simulink model "gm_sampleModel61706_pp_36_1_sub"  (R2023b)
settings: Solver=VariableStepAuto  StartTime=0.0  StopTime=10.0  RelTol=1e-3
libraries: simulink x39, hdlsllib x2
(part 1 of 2)
settings Model: Creator=CW  LastModifiedBy=CW
settings OptimizationCC: BlockReduction=off  ConditionallyExecuteInputs=off
settings DebuggingCC: ArtificialAlgebraicLoopMsg=none  InheritedTsInSrcMsg=none

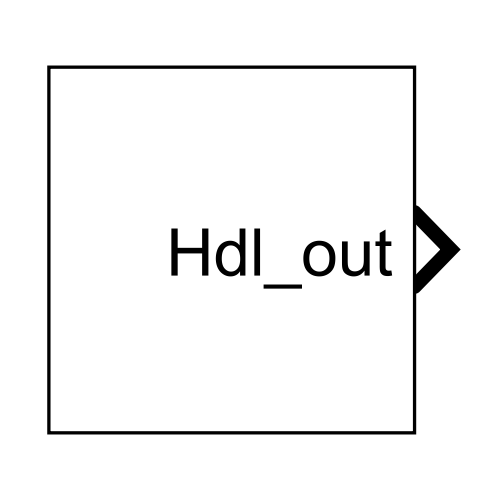
[thumbnail: Simulink's stored preview of the top-level diagram]
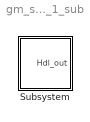
== system gm_sampleModel61706_pp_36_1_sub ==
  Subsystem : Subsystem

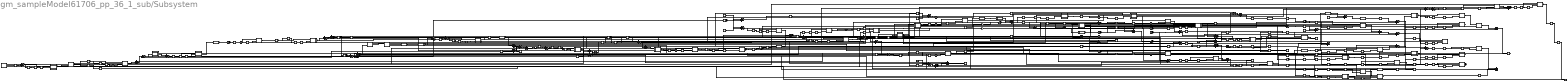
== system gm_sampleModel61706_pp_36_1_sub/Subsystem ==
  Reshape{,1..8} (9 alike) : Reshape
  cfblk1 : Constant  Value=0  OutDataTypeStr=uint8  SampleTime=1
  cfblk10 : Subsystem
  cfblk{11,14..15,20,31,34,39,41,47..48,54,56,58,73,87,90..91,94..95,100,111,118..119,122,125,127,130,133..134,138,141,158,169,178} (34 alike) : Sum  OutDataTypeStr=uint8  AccumDataTypeStr=uint8  SampleTime=1
  cfblk{26,101,110,148,166,168,184} (7 alike) : MinMax  OutDataTypeStr=uint8
  cfblk102 : Subsystem
  cfblk103 : Subsystem
  cfblk{18,42,51,79,84,104,120,132,136,147,153,165} (12 alike) : Product  Inputs=*/  OutDataTypeStr=uint8  RndMeth=Zero  SaturateOnIntegerOverflow=on  SampleTime=1
  cfblk105 : Subsystem
  cfblk106_inst : Subsystem
  cfblk{17,19,40,44,59,62,83,107..108,112,114,159,180,183} (14 alike) : Sum  Inputs=+-  OutDataTypeStr=uint8  AccumDataTypeStr=uint8  SampleTime=1
  cfblk{21,25,52,65,75,93,109,115,124,151,163,167} (12 alike) : Sum  Inputs=+  OutDataTypeStr=uint8
  cfblk{23,29..30,43,53,113} (6 alike) : Gain  Gain="fi(0,0,8,7,\"hex\",\"80\")"  ParamDataTypeStr=fixdt(0, 8, 7)  OutDataTypeStr=uint8  SampleTime=1
  cfblk116 : Subsystem
  cfblk117 : Subsystem
  cfblk12 : Subsystem
  cfblk123 : Subsystem
  cfblk126 : Subsystem
  cfblk129 : Subsystem
  cfblk13 : Subsystem  mask(Real World Value Increment){}
      mask help: Simulink:masks:RealWorldValueIncrement_MD
      mask Display: disp('V++')
  cfblk{24,63,131,142..144,149,152} (8 alike) : Abs  SampleTime=1  OutDataTypeStr=uint8  SaturateOnIntegerOverflow=off
  cfblk{69,92,135,140,160} (5 alike) : Signum  SampleTime=1
  cfblk{27,36,67..68,137,156,170..171,175} (9 alike) : Sum  OutDataTypeStr=uint8  AccumDataTypeStr=uint8  RndMeth=Nearest  SampleTime=1
  cfblk137_const_val : Constant  Value=0  VectorParams1D=off  OutDataTypeStr=uint8  SampleTime=1
  cfblk139_inst : Subsystem
  cfblk145 : Subsystem
  cfblk146_inst : Subsystem
  cfblk150_inst : Subsystem
  cfblk{22,33,78,154} (4 alike) : ComplexToRealImag  SampleTime=1
  cfblk155 : Subsystem
  cfblk156_const_val : Constant  Value=0  VectorParams1D=off  OutDataTypeStr=uint8  SampleTime=1
  cfblk157_inst : Subsystem
  cfblk16 : Subsystem
  cfblk161 : Subsystem
  cfblk162_inst : Subsystem
  cfblk164 : Subsystem
  cfblk170_const_val : Constant  Value=0  VectorParams1D=off  OutDataTypeStr=uint8  SampleTime=1
  cfblk171_const_val : Constant  Value=0  VectorParams1D=off  OutDataTypeStr=uint8  SampleTime=1
  cfblk172_inst : Subsystem
  cfblk174 : Subsystem
  cfblk175_const_val : Constant  Value=0  VectorParams1D=off  OutDataTypeStr=uint8  SampleTime=1
  cfblk176 : Subsystem
  cfblk179 : Subsystem
  cfblk182 : Subsystem  mask(Real World Value Increment){}
      mask help: Simulink:masks:RealWorldValueIncrement_MD
      mask Display: disp('V++')
  cfblk185 : Constant  Value=double(0)  VectorParams1D=off  OutDataTypeStr=double  SampleTime=1
  cfblk186 : hdlsllib/Sources/HDL Counter  CountType=Count limited  CountInit=0  CountStep=1  CountMax=25  CountFromType=Initial value  CountFrom=0  CountResetPort=off  CountLoadPort=off  CountEnbPort=off  CountDirPort=off  CountHitOutputPort=off  CountDataType=Unsigned  CountWordLen=8  CountFracLen=0  CountSampTime=1
  cfblk187 : Constant  OutDataTypeStr=uint8  SampleTime=1
  cfblk188 : Subsystem
  cfblk189 : Subsystem
  cfblk190 : Switch  Threshold=double(0)  OutDataTypeStr=uint8  SampleTime=1  SaturateOnIntegerOverflow=off  InputSameDT=off
  cfblk191 : Switch  Threshold=double(0)  OutDataTypeStr=uint8  SampleTime=1  SaturateOnIntegerOverflow=off  InputSameDT=off
  cfblk192 : Switch  Threshold=double(0)  OutDataTypeStr=uint8  SampleTime=1  SaturateOnIntegerOverflow=off  InputSameDT=off
  cfblk{193..196,198..199,201..215,217} (22 alike) : Delay  DelayLength=double(2)  InitialCondition=0  SampleTime=1
  cfblk197 : Subsystem
  cfblk2 : Subsystem  mask(Compare To Constant){relop=<=, const=double(3), OutDataTypeStr=uint8, ZeroCross=on}
      mask prompts: relop "Simulink:masks:Operator_MP"; const "Simulink:masks:ConstantValue_MP"; OutDataTypeStr "Simulink:masks:OutputDataType_MP"; ZeroCross "Simulink:masks:EnableZerocrossingDetection_MP"
      mask help: Simulink:masks:CompareToConstant_MD
      mask init:
      | OutDataTypeStr = 'uint8';
      | ZeroCross = 'on';
      | blkName = 'sampleModel61706_pp_36_1_sub/Subsystem/cfblk2';
      | const = double(3);
      | const_str = '3.0';
      | const_val = double(3);
      | relop = '<=';
      | setValue = 'fixdt(0, 8)';
      | str = '<= 3';
      mask TypeOptions relop: == | ~= | < | <= | >= | >
      mask TypeOptions OutDataTypeStr: Simulink:masks:uint8 | Simulink:masks:boolean
      mask Callback ZeroCross: sl('zeroCrossEnable', gcbh);
      mask Display: disp(str)
  cfblk200 : Subsystem
  cfblk218 : Subsystem
  cfblk219 : DataTypeConversion  OutDataTypeStr=fixdt(0,8,0)
  cfblk27_const_val : Constant  Value=0  VectorParams1D=off  OutDataTypeStr=uint8  SampleTime=1
  cfblk28 : Subsystem
  cfblk3 : Subsystem
  cfblk32 : Subsystem
  cfblk36_const_val : Constant  Value=0  VectorParams1D=off  OutDataTypeStr=uint8  SampleTime=1
  cfblk37 : Subsystem
  cfblk38 : Subsystem
  cfblk4 : Subsystem  mask(Compare To Zero){relop=<=, OutDataTypeStr=uint8, ZeroCross=on}
      mask prompts: relop "Simulink:masks:Operator_MP"; OutDataTypeStr "Simulink:masks:OutputDataType_MP"; ZeroCross "Simulink:masks:EnableZerocrossingDetection_MP"
      mask help: Simulink:masks:CompareToZero_MD
      mask init:
      | OutDataTypeStr = 'uint8';
      | ZeroCross = 'on';
      | blkName = 'sampleModel61706_pp_36_1_sub/Subsystem/cfblk4';
      | relop = '<=';
      | setValue = 'fixdt(0, 8)';
      mask TypeOptions relop: == | ~= | < | <= | >= | >
      mask TypeOptions OutDataTypeStr: Simulink:masks:uint8 | Simulink:masks:boolean
      mask Callback ZeroCross: sl('zeroCrossEnable', gcbh);
      mask Display: disp([relop,' 0'])
  cfblk45_inst : Subsystem
  cfblk49 : Subsystem
  cfblk5 : Subsystem  mask(Compare To Constant){relop=<=, const=double(3), OutDataTypeStr=uint8, ZeroCross=on}
      mask prompts: relop "Simulink:masks:Operator_MP"; const "Simulink:masks:ConstantValue_MP"; OutDataTypeStr "Simulink:masks:OutputDataType_MP"; ZeroCross "Simulink:masks:EnableZerocrossingDetection_MP"
      mask help: Simulink:masks:CompareToConstant_MD
      mask init:
      | OutDataTypeStr = 'uint8';
      | ZeroCross = 'on';
      | blkName = 'sampleModel61706_pp_36_1_sub/Subsystem/cfblk5';
      | const = double(3);
      | const_str = '3.0';
      | const_val = double(3);
      | relop = '<=';
      | setValue = 'fixdt(0, 8)';
      | str = '<= 3';
      mask TypeOptions relop: == | ~= | < | <= | >= | >
      mask TypeOptions OutDataTypeStr: Simulink:masks:uint8 | Simulink:masks:boolean
      mask Callback ZeroCross: sl('zeroCrossEnable', gcbh);
      mask Display: disp(str)
  cfblk50 : Sum  OutDataTypeStr=uint8  AccumDataTypeStr=fixdt(0, 32, 7)  SampleTime=1
  cfblk55 : Subsystem
  cfblk57 : Subsystem
  cfblk60 : Subsystem  mask(Real World Value Increment){}
      mask help: Simulink:masks:RealWorldValueIncrement_MD
      mask Display: disp('V++')
  cfblk64 : Subsystem
  cfblk66 : Subsystem
  cfblk67_const_val : Constant  Value=0  VectorParams1D=off  OutDataTypeStr=uint8  SampleTime=1
  cfblk68_const_val : Constant  Value=0  VectorParams1D=off  OutDataTypeStr=uint8  SampleTime=1
  cfblk6_inst : Subsystem
  cfblk7 : Subsystem
  cfblk70 : Subsystem  mask(Real World Value Increment){}
      mask help: Simulink:masks:RealWorldValueIncrement_MD
      mask Display: disp('V++')
  cfblk71_inst : Subsystem
  cfblk72 : Subsystem  mask(Real World Value Increment){}
      mask help: Simulink:masks:RealWorldValueIncrement_MD
      mask Display: disp('V++')
  cfblk74 : Subsystem
  cfblk76 : Subsystem
  cfblk77 : Sum  OutDataTypeStr=uint8  AccumDataTypeStr=fixdt(0, 32, 7)  SampleTime=1
  cfblk8 : Subsystem
  cfblk80 : Subsystem  mask(Real World Value Increment){}
      mask help: Simulink:masks:RealWorldValueIncrement_MD
      mask Display: disp('V++')
  cfblk81 : Subsystem  mask(Real World Value Increment){}
      mask help: Simulink:masks:RealWorldValueIncrement_MD
      mask Display: disp('V++')
  cfblk85 : Sum  OutDataTypeStr=uint8  AccumDataTypeStr=fixdt(0, 32, 7)  SampleTime=1
  cfblk86_inst : Subsystem
  cfblk88 : Gain  Gain="fi(0,0,16,15,\"hex\",\"8000\")"  ParamDataTypeStr=fixdt(0, 16, 15)  OutDataTypeStr=uint8  SampleTime=1
  cfblk89 : Subsystem
  cfblk9 : Subsystem  mask(Real World Value Increment){}
      mask help: Simulink:masks:RealWorldValueIncrement_MD
      mask Display: disp('V++')
  cfblk96 : Subsystem
  cfblk97_inst : Subsystem
  cfblk98 : Subsystem
  cfblk99 : Subsystem
  compare{,1,8..11,14,16..19,23,25,27..28,32..37} (21 alike) : simulink/Logic and Bit Operations/Compare To Constant  relop=>=  const=255  OutDataTypeStr=boolean
  compare{2,4..7,12..13,15,20,22,24,26,29..31} (15 alike) : simulink/Logic and Bit Operations/Compare To Constant  relop=>=  const=0  OutDataTypeStr=boolean
  compare21 : simulink/Logic and Bit Operations/Compare To Constant  relop=>=  const=1  OutDataTypeStr=boolean
  compare3 : simulink/Logic and Bit Operations/Compare To Constant  relop=>=  const=1  OutDataTypeStr=boolean
  compare38 : simulink/Logic and Bit Operations/Compare To Constant  relop=>=  const=1  OutDataTypeStr=boolean
  emi_{6,14,22,30,39,47,55,63,71,79,87,95,103,111,119,127,136,144,152,160,176,184,192,200,208,216,224,232,240,256,264,272,280,288,296,304,312} (37 alike) : DataTypeConversion  OutDataTypeStr=fixdt(0,8,0)
  emi_{7,56,64,72,80,88,104,112,161,169,177,185,209,217,225,233,241,273,289,297,305} (21 alike) : Delay  DelayLength=double(2)  InitialCondition=255  SampleTime=1
  emi_{15,23,31,40,48,120,137,145,153,193,201,249,265,281,313} (15 alike) : Delay  DelayLength=double(2)  InitialCondition=0  SampleTime=1
  emi_128 : Delay  DelayLength=double(2)  InitialCondition=1  SampleTime=1
  emi_168 : DataTypeConversion  OutDataTypeStr=uint8  SampleTime=1  SaturateOnIntegerOverflow=off  RndMeth=Floor
  emi_248 : DataTypeConversion  OutDataTypeStr=uint8  SampleTime=1  SaturateOnIntegerOverflow=off  RndMeth=Floor
  emi_257 : Delay  DelayLength=double(2)  InitialCondition=1  SampleTime=1
  emi_96 : Delay  DelayLength=double(2)  InitialCondition=1  SampleTime=1
  Hdl_out : Outport  OutDataTypeStr=uint8  SampleTime=1
  wires:
  cfblk1/1 -> cfblk114/1
  cfblk10/1(emi_2) -> cfblk206/1
  cfblk100/1 -> cfblk22/1, cfblk165/1
  cfblk101/1 -> emi_161/1, cfblk3/1(emi_155)
  cfblk102/1(emi_10) -> cfblk130/1
  cfblk103/1(emi_115) -> cfblk120/1
  cfblk104/1 -> emi_185/1, cfblk38/1(emi_179), cfblk120/2
  cfblk105/1(emi_276) -> cfblk63/1, cfblk34/2
  cfblk106_inst/1(out1) -> cfblk135/1, cfblk25/1
  cfblk107/1 -> cfblk211/1
  cfblk108/1 -> cfblk188/1(In1)
  cfblk109/1 -> cfblk178/2, cfblk134/1
  cfblk11/1 -> emi_104/1, cfblk161/1(emi_98)
  cfblk110/1 -> cfblk41/2, cfblk137/1
  cfblk111/1 -> cfblk100/1, emi_80/1, cfblk145/1(emi_74)
  cfblk112/1 -> cfblk90/1, Hdl_out/1
  cfblk113/1 -> emi_145/1, cfblk218/1(emi_139)
  cfblk114/1 -> cfblk133/1
  cfblk115/1 -> cfblk192/3, emi_201/1, cfblk49/1(emi_195)
  cfblk116/1(emi_18) -> cfblk30/1
  cfblk117/1(emi_26) -> emi_281/1, cfblk105/1(emi_275)
  cfblk118/1 -> cfblk59/1
  cfblk119/1 -> cfblk62/1
  cfblk12/1(emi_34) -> cfblk160/1
  cfblk12/2(emi_35) -> cfblk136/2, cfblk79/2
  cfblk120/1 -> cfblk54/2, emi_88/1, cfblk155/1(emi_82)
  Reshape/1 -> cfblk191/1
  cfblk122/1 -> cfblk169/1
  cfblk123/1(emi_43) -> cfblk142/1
  cfblk124/1 -> cfblk19/1
  cfblk125/1 -> emi_56/1, cfblk126/1(emi_50)
  cfblk126/1(emi_51) -> cfblk50/1
  cfblk127/1 -> cfblk6_inst/1(in1)
  Reshape1/1 -> cfblk67/1
  cfblk129/1(emi_59) -> cfblk111/1
  cfblk13/1(y) -> cfblk154/1
  cfblk130/1 -> emi_40/1, cfblk12/1(emi_33)
  cfblk131/1 -> cfblk189/1(In1)
  cfblk132/1 -> cfblk203/1
  cfblk133/1 -> cfblk71_inst/1(in1), cfblk56/2
  cfblk134/1 -> cfblk107/1
  cfblk135/1 -> emi_112/1, cfblk164/1(emi_106)
  cfblk136/1 -> cfblk208/1, cfblk207/1
  cfblk137/1 -> cfblk209/1
  cfblk138/1 -> emi_225/1, cfblk200/1(emi_219)
  cfblk139_inst/1(out1) -> cfblk182/1(u)
  cfblk14/1 -> emi_193/1, cfblk176/1(emi_187)
  cfblk140/1 -> cfblk56/1, cfblk112/1
  cfblk141/1 -> cfblk36/1, cfblk100/2
  cfblk142/1 -> cfblk83/2, cfblk23/1
  cfblk143/1 -> cfblk150_inst/1(in1), cfblk134/2, cfblk111/2
  cfblk144/1 -> cfblk153/2
  cfblk145/1(emi_75) -> emi_7/1, cfblk10/1(emi_1)
  cfblk146_inst/1(out1) -> emi_273/1, cfblk197/1(emi_267)
  cfblk147/1 -> cfblk85/1, cfblk131/1
  cfblk148/1 -> emi_257/1, cfblk76/1(emi_251)
  cfblk149/1 -> emi_241/1, cfblk7/1(emi_235)
  cfblk15/1 -> emi_15/1, cfblk102/1(emi_9)
  cfblk150_inst/1(out1) -> cfblk166/1
  cfblk151/1 -> cfblk143/1, cfblk108/1
  cfblk152/1 -> cfblk73/1, cfblk41/1, cfblk162_inst/1(in1)
  cfblk153/1 -> cfblk11/1
  cfblk154/1 -> cfblk58/1
  cfblk154/2 -> Reshape2/1, cfblk80/1(u)
  cfblk155/1(emi_83) -> cfblk190/1, cfblk17/1
  cfblk156/1 -> cfblk2/1(u)
  cfblk157_inst/1(out1) -> cfblk44/2, cfblk202/1
  cfblk158/1 -> cfblk21/1
  cfblk159/1 -> cfblk157_inst/2(in2), cfblk204/1
  cfblk16/1(emi_91) -> cfblk77/1
  cfblk160/1 -> cfblk70/1(u)
  cfblk161/1(emi_99) -> cfblk68/1, cfblk17/2
  cfblk162_inst/1(out1) -> cfblk180/1
  cfblk163/1 -> cfblk180/2
  cfblk164/1(emi_107) -> cfblk119/2
  cfblk165/1 -> cfblk59/2
  cfblk166/1 -> cfblk91/1, cfblk26/1
  cfblk167/1 -> cfblk152/1, cfblk42/2
  cfblk168/1 -> cfblk39/1
  cfblk169/1 -> cfblk171/1
  cfblk17/1 -> cfblk192/2
  cfblk170/1 -> cfblk79/1
  cfblk171/1 -> cfblk115/1
  cfblk172_inst/1(out1) -> cfblk139_inst/1(in1)
  Reshape2/1 -> emi_120/1, cfblk103/1(emi_114)
  cfblk174/1(emi_123) -> cfblk47/1
  cfblk175/1 -> Reshape/1
  cfblk176/1(emi_188) -> cfblk95/1
  Reshape3/1 -> cfblk110/1
  cfblk178/1 -> emi_31/1, cfblk117/1(emi_25), cfblk124/1
  cfblk179/1(emi_131) -> Reshape5/1
  cfblk179/2(emi_132) -> cfblk146_inst/1(in1), cfblk198/1
  cfblk18/1 -> cfblk45_inst/1(in1), cfblk93/1
  cfblk180/1 -> emi_217/1, cfblk57/1(emi_211)
  Reshape4/1 -> emi_23/1, cfblk53/1, cfblk116/1(emi_17)
  cfblk182/1(y) -> cfblk81/1(u)
  cfblk183/1 -> emi_48/1, cfblk123/1(emi_42)
  cfblk184/1 -> emi_289/1, cfblk89/1(emi_283)
  cfblk185/1 -> cfblk72/1(u)
  cfblk186/1 -> cfblk50/2, cfblk183/1, cfblk14/1
  cfblk187/1 -> Reshape7/1, cfblk107/2
  cfblk188/1(Out1) -> cfblk125/2, cfblk212/1
  cfblk189/1(Out1) -> cfblk94/2
  cfblk19/1 -> cfblk151/1
  cfblk190/1 -> cfblk122/2, emi_137/1, cfblk199/1, cfblk179/1(emi_130)
  cfblk191/1 -> cfblk158/1
  cfblk192/1 -> cfblk194/1
  cfblk193/1 -> cfblk119/1
  cfblk194/1 -> cfblk51/2
  cfblk195/1 -> cfblk191/3
  cfblk196/1 -> cfblk62/2
  cfblk197/1(emi_268) -> cfblk158/2
  cfblk198/1 -> cfblk114/2
  cfblk199/1 -> cfblk87/2
  cfblk2/1(y) -> cfblk69/1
  cfblk20/1 -> cfblk165/2, cfblk148/1
  cfblk200/1(emi_220) -> cfblk190/3
  cfblk201/1 -> cfblk84/2
  cfblk202/1 -> cfblk150_inst/2(in2)
  cfblk203/1 -> cfblk127/1
  cfblk204/1 -> cfblk130/2
  cfblk205/1 -> cfblk18/1
  cfblk206/1 -> cfblk85/2
  cfblk207/1 -> cfblk19/2
  cfblk208/1 -> cfblk71_inst/2(in2)
  cfblk209/1 -> cfblk191/2
  cfblk21/1 -> cfblk5/1(u)
  cfblk210/1 -> cfblk15/2
  cfblk211/1 -> cfblk122/1
  cfblk212/1 -> cfblk106_inst/1(in1)
  cfblk213/1 -> cfblk31/2
  cfblk214/1 -> cfblk169/2
  cfblk215/1 -> cfblk147/2
  cfblk217/1 -> cfblk133/2
  cfblk218/1(emi_140) -> cfblk31/1, cfblk172_inst/1(in1)
  cfblk219/1 -> cfblk113/1
  cfblk22/1 -> cfblk140/1
  cfblk22/2 -> cfblk92/1
  cfblk23/1 -> emi_153/1, cfblk43/1, cfblk64/1(emi_147)
  cfblk24/1 -> cfblk75/1
  cfblk25/1 -> cfblk217/1
  cfblk26/1 -> cfblk91/2, cfblk20/2
  cfblk27/1 -> cfblk108/2, emi_177/1, cfblk37/1(emi_171)
  cfblk28/1(emi_67) -> cfblk215/1, cfblk104/1
  cfblk29/1 -> cfblk109/1
  cfblk3/1(emi_156) -> cfblk159/2, cfblk141/2
  cfblk30/1 -> cfblk9/1(u)
  cfblk31/1 -> cfblk15/1
  cfblk32/1(emi_164) -> cfblk88/1
  cfblk33/1 -> cfblk147/1
  cfblk33/2 -> cfblk13/1(u)
  cfblk34/1 -> emi_64/1, cfblk129/1(emi_58)
  Reshape5/1 -> cfblk48/2, cfblk170/1
  cfblk36/1 -> cfblk138/2, cfblk118/2
  cfblk37/1(emi_172) -> cfblk94/1
  cfblk38/1(emi_180) -> cfblk58/2
  cfblk39/1 -> cfblk153/1
  cfblk4/1(y) -> cfblk178/1
  cfblk40/1 -> cfblk193/1
  cfblk41/1 -> cfblk95/2, cfblk44/1
  cfblk42/1 -> cfblk138/1, emi_305/1, cfblk210/1, cfblk98/1(emi_299)
  cfblk43/1 -> emi_265/1, cfblk8/1(emi_259)
  cfblk44/1 -> cfblk201/1
  cfblk45_inst/1(out1) -> emi_297/1, cfblk96/1(emi_291)
  Reshape6/1 -> cfblk136/1, cfblk52/1
  cfblk47/1 -> cfblk90/2
  cfblk48/1 -> cfblk118/1, cfblk196/1
  cfblk49/1(emi_196) -> Reshape8/1, cfblk14/2, cfblk139_inst/2(in2)
  cfblk5/1(y) -> cfblk219/1
  cfblk50/1 -> cfblk213/1
  cfblk51/1 -> cfblk146_inst/2(in2), cfblk125/1, cfblk18/2
  cfblk52/1 -> cfblk47/2
  cfblk53/1 -> cfblk104/2
  cfblk54/1 -> cfblk34/1
  cfblk55/1(emi_204) -> emi_72/1, cfblk28/1(emi_66)
  cfblk56/1 -> cfblk205/1
  cfblk57/1(emi_212) -> cfblk60/1(u)
  cfblk58/1 -> cfblk45_inst/2(in2), cfblk184/1
  cfblk59/1 -> cfblk144/1
  cfblk6_inst/1(out1) -> emi_209/1, cfblk55/1(emi_203)
  cfblk60/1(y) -> cfblk54/1, cfblk149/1
  Reshape7/1 -> emi_96/1, cfblk16/1(emi_90)
  cfblk62/1 -> cfblk162_inst/2(in2), cfblk65/1
  cfblk63/1 -> emi_313/1, cfblk99/1(emi_307)
  cfblk64/1(emi_148) -> emi_249/1, cfblk74/1(emi_243)
  cfblk65/1 -> cfblk27/1, cfblk175/1
  cfblk66/1(emi_228) -> cfblk97_inst/2(in2), cfblk106_inst/2(in2)
  cfblk67/1 -> cfblk40/2, cfblk39/2
  cfblk68/1 -> cfblk192/1
  cfblk69/1 -> cfblk20/1
  cfblk7/1(emi_236) -> cfblk101/1
  cfblk70/1(y) -> cfblk48/1, cfblk51/1
  cfblk71_inst/1(out1) -> cfblk33/1, Reshape4/1
  cfblk72/1(y) -> cfblk4/1(u)
  cfblk73/1 -> Reshape3/1
  cfblk74/1(emi_244) -> cfblk77/2
  cfblk75/1 -> cfblk157_inst/1(in1)
  cfblk76/1(emi_252) -> cfblk141/1
  cfblk77/1 -> emi_128/1, cfblk174/1(emi_122)
  cfblk78/1 -> cfblk168/1
  cfblk78/2 -> cfblk24/1, cfblk132/2
  cfblk79/1 -> cfblk195/1
  cfblk8/1(emi_260) -> cfblk97_inst/1(in1)
  cfblk80/1(y) -> cfblk156/1
  cfblk81/1(y) -> cfblk159/1, cfblk132/1
  Reshape8/1 -> cfblk29/1
  cfblk83/1 -> Reshape1/1
  cfblk84/1 -> cfblk78/1
  cfblk85/1 -> emi_233/1, cfblk66/1(emi_227)
  cfblk86_inst/1(out1) -> cfblk40/1
  cfblk87/1 -> cfblk127/2
  cfblk88/1 -> cfblk83/1
  cfblk89/1(emi_284) -> cfblk190/2
  cfblk9/1(y) -> cfblk163/1
  cfblk90/1 -> cfblk172_inst/2(in2), cfblk84/1
  cfblk91/1 -> cfblk167/1
  cfblk92/1 -> cfblk86_inst/2(in2)
  cfblk93/1 -> cfblk87/1, cfblk73/2, cfblk11/2
  cfblk94/1 -> cfblk6_inst/2(in2), cfblk42/1
  cfblk95/1 -> Reshape6/1
  cfblk96/1(emi_292) -> cfblk86_inst/1(in1)
  cfblk97_inst/1(out1) -> cfblk112/2
  cfblk98/1(emi_300) -> emi_169/1, cfblk32/1(emi_163)
  cfblk99/1(emi_308) -> cfblk183/2, cfblk214/1
  emi_103/1 -> compare/1
  emi_104/1 -> emi_103/1
  emi_111/1 -> compare1/1
  emi_112/1 -> emi_111/1
  emi_119/1 -> compare2/1
  emi_120/1 -> emi_119/1
  emi_127/1 -> compare3/1
  emi_128/1 -> emi_127/1
  emi_136/1 -> compare5/1
  emi_137/1 -> emi_136/1
  emi_14/1 -> compare4/1
  emi_144/1 -> compare6/1
  emi_145/1 -> emi_144/1
  emi_15/1 -> emi_14/1
  emi_152/1 -> compare7/1
  emi_153/1 -> emi_152/1
  emi_160/1 -> compare8/1
  emi_161/1 -> emi_160/1
  emi_168/1 -> compare9/1
  emi_169/1 -> emi_168/1
  emi_176/1 -> compare10/1
  emi_177/1 -> emi_176/1
  emi_184/1 -> compare11/1
  emi_185/1 -> emi_184/1
  emi_192/1 -> compare12/1
  emi_193/1 -> emi_192/1
  emi_200/1 -> compare13/1
  emi_201/1 -> emi_200/1
  emi_208/1 -> compare14/1
  emi_209/1 -> emi_208/1
  emi_216/1 -> compare16/1
  emi_217/1 -> emi_216/1
  emi_22/1 -> compare15/1
  emi_224/1 -> compare17/1
  emi_225/1 -> emi_224/1
  emi_23/1 -> emi_22/1
  emi_232/1 -> compare18/1
  emi_233/1 -> emi_232/1
  emi_240/1 -> compare19/1
  emi_241/1 -> emi_240/1
  emi_248/1 -> compare20/1
  emi_249/1 -> emi_248/1
  emi_256/1 -> compare21/1
  emi_257/1 -> emi_256/1
  emi_264/1 -> compare22/1
  emi_265/1 -> emi_264/1
  emi_272/1 -> compare23/1
  emi_273/1 -> emi_272/1
  emi_280/1 -> compare24/1
  emi_281/1 -> emi_280/1
  emi_288/1 -> compare25/1
  emi_289/1 -> emi_288/1
  emi_296/1 -> compare27/1
  emi_297/1 -> emi_296/1
  emi_30/1 -> compare26/1
  emi_304/1 -> compare28/1
  emi_305/1 -> emi_304/1
  emi_31/1 -> emi_30/1
  emi_312/1 -> compare29/1
  emi_313/1 -> emi_312/1
  emi_39/1 -> compare30/1
  emi_40/1 -> emi_39/1
  emi_47/1 -> compare31/1
  emi_48/1 -> emi_47/1
  emi_55/1 -> compare33/1
  emi_56/1 -> emi_55/1
  emi_6/1 -> compare32/1
  emi_63/1 -> compare34/1
  emi_64/1 -> emi_63/1
  emi_7/1 -> emi_6/1
  emi_71/1 -> compare35/1
  emi_72/1 -> emi_71/1
  emi_79/1 -> compare36/1
  emi_80/1 -> emi_79/1
  emi_87/1 -> compare37/1
  emi_88/1 -> emi_87/1
  emi_95/1 -> compare38/1
  emi_96/1 -> emi_95/1
  cfblk137_const_val/1 -> cfblk137/2
  cfblk156_const_val/1 -> cfblk156/2
  cfblk170_const_val/1 -> cfblk170/2
  cfblk171_const_val/1 -> cfblk171/2
  cfblk175_const_val/1 -> cfblk175/2
  cfblk27_const_val/1 -> cfblk27/2
  cfblk36_const_val/1 -> cfblk36/2
  cfblk67_const_val/1 -> cfblk67/2
  cfblk68_const_val/1 -> cfblk68/2
  compare/1 -> cfblk161/2(Action Port)
  compare1/1 -> cfblk164/2(Action Port)
  compare2/1 -> cfblk103/2(Action Port)
  compare3/1 -> cfblk174/2(Action Port)
  compare4/1 -> cfblk102/2(Action Port)
  compare5/1 -> cfblk179/2(Action Port)
  compare6/1 -> cfblk218/2(Action Port)
  compare7/1 -> cfblk64/2(Action Port)
  compare8/1 -> cfblk3/2(Action Port)
  compare9/1 -> cfblk32/2(Action Port)
  compare10/1 -> cfblk37/2(Action Port)
  compare11/1 -> cfblk38/2(Action Port)
  compare12/1 -> cfblk176/2(Action Port)
  compare13/1 -> cfblk49/2(Action Port)
  compare14/1 -> cfblk55/2(Action Port)
  compare15/1 -> cfblk116/2(Action Port)
  compare16/1 -> cfblk57/2(Action Port)
  compare17/1 -> cfblk200/2(Action Port)
  compare18/1 -> cfblk66/2(Action Port)
  compare19/1 -> cfblk7/2(Action Port)
  compare20/1 -> cfblk74/2(Action Port)
  compare21/1 -> cfblk76/2(Action Port)
  compare22/1 -> cfblk8/2(Action Port)
  compare23/1 -> cfblk197/2(Action Port)
  compare24/1 -> cfblk105/2(Action Port)
  compare25/1 -> cfblk89/2(Action Port)
  compare26/1 -> cfblk117/2(Action Port)
  compare27/1 -> cfblk96/2(Action Port)
  compare28/1 -> cfblk98/2(Action Port)
  compare29/1 -> cfblk99/2(Action Port)
  compare30/1 -> cfblk12/2(Action Port)
  compare31/1 -> cfblk123/2(Action Port)
  compare32/1 -> cfblk10/2(Action Port)
  compare33/1 -> cfblk126/2(Action Port)
  compare34/1 -> cfblk129/2(Action Port)
  compare35/1 -> cfblk28/2(Action Port)
  compare36/1 -> cfblk145/2(Action Port)
  compare37/1 -> cfblk155/2(Action Port)
  compare38/1 -> cfblk16/2(Action Port)

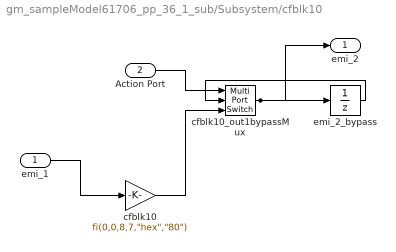
== system gm_sampleModel61706_pp_36_1_sub/Subsystem/cfblk10 ==
  emi_1 : Inport  OutDataTypeStr=uint8  PortDimensions=1  SampleTime=1
  Action Port : Inport  Port=2  OutDataTypeStr=boolean  SampleTime=1
  cfblk10 : Gain  Gain="fi(0,0,8,7,\"hex\",\"80\")"  ParamDataTypeStr=fixdt(0, 8, 7)  OutDataTypeStr=fixdt(0, 16, 7)  SampleTime=1
  cfblk10_out1bypassMux : MultiPortSwitch  DataPortOrder=Zero-based contiguous  Inputs=2  zeroidx=on  OutDataTypeStr=fixdt(0, 16, 7)  SampleTime=1  SaturateOnIntegerOverflow=off  InputSameDT=off
  emi_2_bypass : UnitDelay  InitialCondition="fi(0,0,16,7,\"hex\",\"0000\")"  SampleTime=1
  emi_2 : Outport  SampleTime=1  InitialOutput=0
  wires:
  Action Port/1 -> cfblk10_out1bypassMux/1
  emi_1/1 -> cfblk10/1
  cfblk10/1 -> cfblk10_out1bypassMux/3
  cfblk10_out1bypassMux/1 -> emi_2_bypass/1, emi_2/1
  emi_2_bypass/1 -> cfblk10_out1bypassMux/2

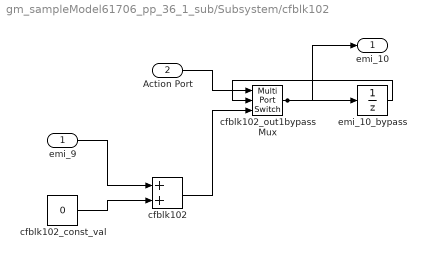
== system gm_sampleModel61706_pp_36_1_sub/Subsystem/cfblk102 ==
  emi_9 : Inport  OutDataTypeStr=uint8  PortDimensions=1  SampleTime=1
  Action Port : Inport  Port=2  OutDataTypeStr=boolean  SampleTime=1
  cfblk102 : Sum  OutDataTypeStr=uint8  AccumDataTypeStr=uint8  RndMeth=Nearest  SampleTime=1
  cfblk102_const_val : Constant  Value=0  VectorParams1D=off  OutDataTypeStr=uint8  SampleTime=1
  cfblk102_out1bypassMux : MultiPortSwitch  DataPortOrder=Zero-based contiguous  Inputs=2  zeroidx=on  OutDataTypeStr=uint8  SampleTime=1  SaturateOnIntegerOverflow=off  InputSameDT=off
  emi_10_bypass : UnitDelay  InitialCondition="fi(0,0,8,0,\"hex\",\"00\")"  SampleTime=1
  emi_10 : Outport  SampleTime=1  InitialOutput=0
  wires:
  Action Port/1 -> cfblk102_out1bypassMux/1
  emi_9/1 -> cfblk102/1
  cfblk102/1 -> cfblk102_out1bypassMux/3
  cfblk102_out1bypassMux/1 -> emi_10_bypass/1, emi_10/1
  emi_10_bypass/1 -> cfblk102_out1bypassMux/2
  cfblk102_const_val/1 -> cfblk102/2

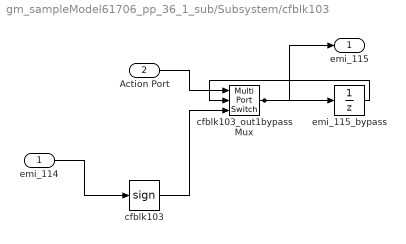
== system gm_sampleModel61706_pp_36_1_sub/Subsystem/cfblk103 ==
  emi_114 : Inport  OutDataTypeStr=uint8  PortDimensions=1  SampleTime=1
  Action Port : Inport  Port=2  OutDataTypeStr=boolean  SampleTime=1
  cfblk103 : Signum  SampleTime=1
  cfblk103_out1bypassMux : MultiPortSwitch  DataPortOrder=Zero-based contiguous  Inputs=2  zeroidx=on  OutDataTypeStr=uint8  SampleTime=1  SaturateOnIntegerOverflow=off  InputSameDT=off
  emi_115_bypass : UnitDelay  InitialCondition="fi(0,0,8,0,\"hex\",\"00\")"  SampleTime=1
  emi_115 : Outport  SampleTime=1  InitialOutput=0
  wires:
  Action Port/1 -> cfblk103_out1bypassMux/1
  emi_114/1 -> cfblk103/1
  cfblk103/1 -> cfblk103_out1bypassMux/3
  cfblk103_out1bypassMux/1 -> emi_115_bypass/1, emi_115/1
  emi_115_bypass/1 -> cfblk103_out1bypassMux/2

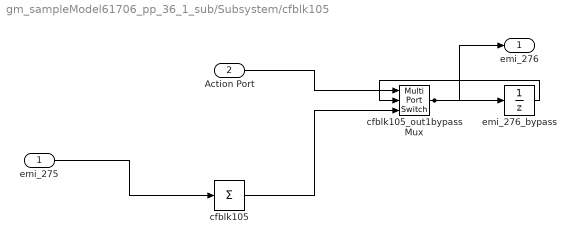
== system gm_sampleModel61706_pp_36_1_sub/Subsystem/cfblk105 ==
  emi_275 : Inport  OutDataTypeStr=uint8  PortDimensions=1  SampleTime=1
  Action Port : Inport  Port=2  OutDataTypeStr=boolean  SampleTime=1
  cfblk105 : Sum  Inputs=+
  cfblk105_out1bypassMux : MultiPortSwitch  DataPortOrder=Zero-based contiguous  Inputs=2  zeroidx=on  OutDataTypeStr=uint8  SampleTime=1  SaturateOnIntegerOverflow=off  InputSameDT=off
  emi_276_bypass : UnitDelay  InitialCondition="fi(0,0,8,0,\"hex\",\"00\")"  SampleTime=1
  emi_276 : Outport  SampleTime=1  InitialOutput=0
  wires:
  Action Port/1 -> cfblk105_out1bypassMux/1
  emi_275/1 -> cfblk105/1
  cfblk105/1 -> cfblk105_out1bypassMux/3
  cfblk105_out1bypassMux/1 -> emi_276_bypass/1, emi_276/1
  emi_276_bypass/1 -> cfblk105_out1bypassMux/2

== system gm_sampleModel61706_pp_36_1_sub/Subsystem/cfblk106_inst ==
  in1 : Inport  OutDataTypeStr=uint8  SampleTime=1
  in2 : Inport  Port=2  OutDataTypeStr=uint8  SampleTime=1
  mul_cfblk106_dotp_mulcomp : Product  Inputs=**  OutDataTypeStr=uint8  SampleTime=1
  out1 : Outport  OutDataTypeStr=uint8  SampleTime=1
  wires:
  in1/1 -> mul_cfblk106_dotp_mulcomp/1
  in2/1 -> mul_cfblk106_dotp_mulcomp/2
  mul_cfblk106_dotp_mulcomp/1 -> out1/1

== system gm_sampleModel61706_pp_36_1_sub/Subsystem/cfblk116 ==
  emi_17 : Inport  OutDataTypeStr=uint8  PortDimensions=1  SampleTime=1
  Action Port : Inport  Port=2  OutDataTypeStr=boolean  SampleTime=1
  Reshape : Reshape
  cfblk116_out1bypassMux : MultiPortSwitch  DataPortOrder=Zero-based contiguous  Inputs=2  zeroidx=on  OutDataTypeStr=uint8  SampleTime=1  SaturateOnIntegerOverflow=off  InputSameDT=off
  emi_18_bypass : UnitDelay  InitialCondition="fi(0,0,8,0,\"hex\",\"00\")"  SampleTime=1
  emi_18 : Outport  SampleTime=1  InitialOutput=0
  wires:
  Action Port/1 -> cfblk116_out1bypassMux/1
  emi_17/1 -> Reshape/1
  Reshape/1 -> cfblk116_out1bypassMux/3
  cfblk116_out1bypassMux/1 -> emi_18_bypass/1, emi_18/1
  emi_18_bypass/1 -> cfblk116_out1bypassMux/2

== system gm_sampleModel61706_pp_36_1_sub/Subsystem/cfblk117 ==
  emi_25 : Inport  OutDataTypeStr=uint8  PortDimensions=1  SampleTime=1
  Action Port : Inport  Port=2  OutDataTypeStr=boolean  SampleTime=1
  cfblk117 : Abs  SampleTime=1  OutDataTypeStr=uint8  SaturateOnIntegerOverflow=off
  cfblk117_out1bypassMux : MultiPortSwitch  DataPortOrder=Zero-based contiguous  Inputs=2  zeroidx=on  OutDataTypeStr=uint8  SampleTime=1  SaturateOnIntegerOverflow=off  InputSameDT=off
  emi_26_bypass : UnitDelay  InitialCondition="fi(0,0,8,0,\"hex\",\"00\")"  SampleTime=1
  emi_26 : Outport  SampleTime=1  InitialOutput=0
  wires:
  Action Port/1 -> cfblk117_out1bypassMux/1
  emi_25/1 -> cfblk117/1
  cfblk117/1 -> cfblk117_out1bypassMux/3
  cfblk117_out1bypassMux/1 -> emi_26_bypass/1, emi_26/1
  emi_26_bypass/1 -> cfblk117_out1bypassMux/2

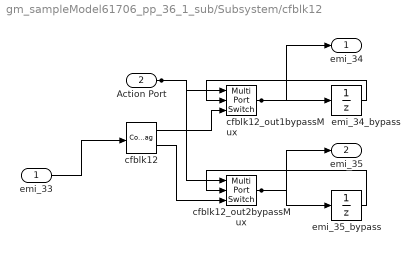
== system gm_sampleModel61706_pp_36_1_sub/Subsystem/cfblk12 ==
  emi_33 : Inport  OutDataTypeStr=uint8  PortDimensions=1  SampleTime=1
  Action Port : Inport  Port=2  OutDataTypeStr=boolean  SampleTime=1
  cfblk12 : ComplexToRealImag  SampleTime=1
  cfblk12_out1bypassMux : MultiPortSwitch  DataPortOrder=Zero-based contiguous  Inputs=2  zeroidx=on  OutDataTypeStr=uint8  SampleTime=1  SaturateOnIntegerOverflow=off  InputSameDT=off
  cfblk12_out2bypassMux : MultiPortSwitch  DataPortOrder=Zero-based contiguous  Inputs=2  zeroidx=on  OutDataTypeStr=uint8  SampleTime=1  SaturateOnIntegerOverflow=off  InputSameDT=off
  emi_34_bypass : UnitDelay  InitialCondition="fi(0,0,8,0,\"hex\",\"00\")"  SampleTime=1
  emi_35_bypass : UnitDelay  InitialCondition="fi(0,0,8,0,\"hex\",\"00\")"  SampleTime=1
  emi_34 : Outport  SampleTime=1  InitialOutput=0
  emi_35 : Outport  Port=2  SampleTime=1  InitialOutput=0
  wires:
  Action Port/1 -> cfblk12_out2bypassMux/1, cfblk12_out1bypassMux/1
  emi_33/1 -> cfblk12/1
  cfblk12/1 -> cfblk12_out1bypassMux/3
  cfblk12/2 -> cfblk12_out2bypassMux/3
  cfblk12_out1bypassMux/1 -> emi_34_bypass/1, emi_34/1
  emi_34_bypass/1 -> cfblk12_out1bypassMux/2
  cfblk12_out2bypassMux/1 -> emi_35_bypass/1, emi_35/1
  emi_35_bypass/1 -> cfblk12_out2bypassMux/2

== system gm_sampleModel61706_pp_36_1_sub/Subsystem/cfblk123 ==
  emi_42 : Inport  OutDataTypeStr=uint8  PortDimensions=1  SampleTime=1
  Action Port : Inport  Port=2  OutDataTypeStr=boolean  SampleTime=1
  cfblk123 : Sum  Inputs=+
  cfblk123_out1bypassMux : MultiPortSwitch  DataPortOrder=Zero-based contiguous  Inputs=2  zeroidx=on  OutDataTypeStr=uint8  SampleTime=1  SaturateOnIntegerOverflow=off  InputSameDT=off
  emi_43_bypass : UnitDelay  InitialCondition="fi(0,0,8,0,\"hex\",\"00\")"  SampleTime=1
  emi_43 : Outport  SampleTime=1  InitialOutput=0
  wires:
  Action Port/1 -> cfblk123_out1bypassMux/1
  emi_42/1 -> cfblk123/1
  cfblk123/1 -> cfblk123_out1bypassMux/3
  cfblk123_out1bypassMux/1 -> emi_43_bypass/1, emi_43/1
  emi_43_bypass/1 -> cfblk123_out1bypassMux/2

== system gm_sampleModel61706_pp_36_1_sub/Subsystem/cfblk126 ==
  emi_50 : Inport  OutDataTypeStr=uint8  PortDimensions=1  SampleTime=1
  Action Port : Inport  Port=2  OutDataTypeStr=boolean  SampleTime=1
  cfblk126 : Gain  Gain="fi(0,0,8,7,\"hex\",\"80\")"  ParamDataTypeStr=fixdt(0, 8, 7)  OutDataTypeStr=fixdt(0, 16, 7)  SampleTime=1
  cfblk126_out1bypassMux : MultiPortSwitch  DataPortOrder=Zero-based contiguous  Inputs=2  zeroidx=on  OutDataTypeStr=fixdt(0, 16, 7)  SampleTime=1  SaturateOnIntegerOverflow=off  InputSameDT=off
  emi_51_bypass : UnitDelay  InitialCondition="fi(0,0,16,7,\"hex\",\"0000\")"  SampleTime=1
  emi_51 : Outport  SampleTime=1  InitialOutput=0
  wires:
  Action Port/1 -> cfblk126_out1bypassMux/1
  emi_50/1 -> cfblk126/1
  cfblk126/1 -> cfblk126_out1bypassMux/3
  cfblk126_out1bypassMux/1 -> emi_51_bypass/1, emi_51/1
  emi_51_bypass/1 -> cfblk126_out1bypassMux/2

== system gm_sampleModel61706_pp_36_1_sub/Subsystem/cfblk129 ==
  emi_58 : Inport  OutDataTypeStr=uint8  PortDimensions=1  SampleTime=1
  Action Port : Inport  Port=2  OutDataTypeStr=boolean  SampleTime=1
  cfblk129 : MinMax
  cfblk129_out1bypassMux : MultiPortSwitch  DataPortOrder=Zero-based contiguous  Inputs=2  zeroidx=on  OutDataTypeStr=uint8  SampleTime=1  SaturateOnIntegerOverflow=off  InputSameDT=off
  emi_59_bypass : UnitDelay  InitialCondition="fi(0,0,8,0,\"hex\",\"00\")"  SampleTime=1
  emi_59 : Outport  SampleTime=1  InitialOutput=0
  wires:
  Action Port/1 -> cfblk129_out1bypassMux/1
  emi_58/1 -> cfblk129/1
  cfblk129/1 -> cfblk129_out1bypassMux/3
  cfblk129_out1bypassMux/1 -> emi_59_bypass/1, emi_59/1
  emi_59_bypass/1 -> cfblk129_out1bypassMux/2

== system gm_sampleModel61706_pp_36_1_sub/Subsystem/cfblk13 ==
  u : Inport  OutDataTypeStr=uint8  SampleTime=1
  FixPt Constant : Constant  DisableCoverage=on  OutDataTypeStr=Inherit: Inherit via back propagation  SampleTime=-1
  FixPt Data Type Duplicate : DataTypeDuplicate  DisableCoverage=on  NumInputPorts=3
  FixPt Sum1 : Sum  OutDataTypeStr=Inherit: Inherit via back propagation  InputSameDT=on  LockScale=on
  y : Outport  SampleTime=1
  wires:
  u/1 -> FixPt Sum1/1, FixPt Data Type Duplicate/2
  FixPt Constant/1 -> FixPt Sum1/2, FixPt Data Type Duplicate/3
  FixPt Sum1/1 -> FixPt Data Type Duplicate/1, y/1

== system gm_sampleModel61706_pp_36_1_sub/Subsystem/cfblk139_inst ==
  in1 : Inport  OutDataTypeStr=uint8  SampleTime=1
  in2 : Inport  Port=2  OutDataTypeStr=uint8  SampleTime=1
  mul_cfblk139_dotp_mulcomp : Product  Inputs=**  OutDataTypeStr=uint8  SampleTime=1
  out1 : Outport  OutDataTypeStr=uint8  SampleTime=1
  wires:
  in1/1 -> mul_cfblk139_dotp_mulcomp/1
  in2/1 -> mul_cfblk139_dotp_mulcomp/2
  mul_cfblk139_dotp_mulcomp/1 -> out1/1

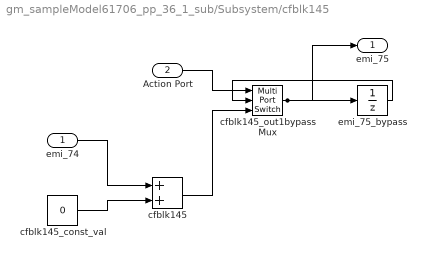
== system gm_sampleModel61706_pp_36_1_sub/Subsystem/cfblk145 ==
  emi_74 : Inport  OutDataTypeStr=uint8  PortDimensions=1  SampleTime=1
  Action Port : Inport  Port=2  OutDataTypeStr=boolean  SampleTime=1
  cfblk145 : Sum  OutDataTypeStr=uint8  AccumDataTypeStr=uint8  RndMeth=Nearest  SampleTime=1
  cfblk145_const_val : Constant  Value=0  VectorParams1D=off  OutDataTypeStr=uint8  SampleTime=1
  cfblk145_out1bypassMux : MultiPortSwitch  DataPortOrder=Zero-based contiguous  Inputs=2  zeroidx=on  OutDataTypeStr=uint8  SampleTime=1  SaturateOnIntegerOverflow=off  InputSameDT=off
  emi_75_bypass : UnitDelay  InitialCondition="fi(0,0,8,0,\"hex\",\"00\")"  SampleTime=1
  emi_75 : Outport  SampleTime=1  InitialOutput=0
  wires:
  Action Port/1 -> cfblk145_out1bypassMux/1
  emi_74/1 -> cfblk145/1
  cfblk145/1 -> cfblk145_out1bypassMux/3
  cfblk145_out1bypassMux/1 -> emi_75_bypass/1, emi_75/1
  emi_75_bypass/1 -> cfblk145_out1bypassMux/2
  cfblk145_const_val/1 -> cfblk145/2

== system gm_sampleModel61706_pp_36_1_sub/Subsystem/cfblk146_inst ==
  in1 : Inport  OutDataTypeStr=uint8  SampleTime=1
  in2 : Inport  Port=2  OutDataTypeStr=uint8  SampleTime=1
  mul_cfblk146_dotp_mulcomp : Product  Inputs=**  OutDataTypeStr=uint8  SampleTime=1
  out1 : Outport  OutDataTypeStr=uint8  SampleTime=1
  wires:
  in1/1 -> mul_cfblk146_dotp_mulcomp/1
  in2/1 -> mul_cfblk146_dotp_mulcomp/2
  mul_cfblk146_dotp_mulcomp/1 -> out1/1

== system gm_sampleModel61706_pp_36_1_sub/Subsystem/cfblk150_inst ==
  in1 : Inport  OutDataTypeStr=uint8  SampleTime=1
  in2 : Inport  Port=2  OutDataTypeStr=uint8  SampleTime=1
  mul_cfblk150_dotp_mulcomp : Product  Inputs=**  OutDataTypeStr=uint8  SampleTime=1
  out1 : Outport  OutDataTypeStr=uint8  SampleTime=1
  wires:
  in1/1 -> mul_cfblk150_dotp_mulcomp/1
  in2/1 -> mul_cfblk150_dotp_mulcomp/2
  mul_cfblk150_dotp_mulcomp/1 -> out1/1

== system gm_sampleModel61706_pp_36_1_sub/Subsystem/cfblk155 ==
  emi_82 : Inport  OutDataTypeStr=uint8  PortDimensions=1  SampleTime=1
  Action Port : Inport  Port=2  OutDataTypeStr=boolean  SampleTime=1
  cfblk155 : Signum  SampleTime=1
  cfblk155_out1bypassMux : MultiPortSwitch  DataPortOrder=Zero-based contiguous  Inputs=2  zeroidx=on  OutDataTypeStr=uint8  SampleTime=1  SaturateOnIntegerOverflow=off  InputSameDT=off
  emi_83_bypass : UnitDelay  InitialCondition="fi(0,0,8,0,\"hex\",\"00\")"  SampleTime=1
  emi_83 : Outport  SampleTime=1  InitialOutput=0
  wires:
  Action Port/1 -> cfblk155_out1bypassMux/1
  emi_82/1 -> cfblk155/1
  cfblk155/1 -> cfblk155_out1bypassMux/3
  cfblk155_out1bypassMux/1 -> emi_83_bypass/1, emi_83/1
  emi_83_bypass/1 -> cfblk155_out1bypassMux/2

== system gm_sampleModel61706_pp_36_1_sub/Subsystem/cfblk157_inst ==
  in1 : Inport  OutDataTypeStr=uint8  SampleTime=1
  in2 : Inport  Port=2  OutDataTypeStr=uint8  SampleTime=1
  mul_cfblk157_dotp_mulcomp : Product  Inputs=**  OutDataTypeStr=uint8  SampleTime=1
  out1 : Outport  OutDataTypeStr=uint8  SampleTime=1
  wires:
  in1/1 -> mul_cfblk157_dotp_mulcomp/1
  in2/1 -> mul_cfblk157_dotp_mulcomp/2
  mul_cfblk157_dotp_mulcomp/1 -> out1/1

== system gm_sampleModel61706_pp_36_1_sub/Subsystem/cfblk16 ==
  emi_90 : Inport  OutDataTypeStr=uint8  PortDimensions=1  SampleTime=1
  Action Port : Inport  Port=2  OutDataTypeStr=boolean  SampleTime=1
  cfblk16 : Gain  Gain="fi(0,0,8,7,\"hex\",\"80\")"  ParamDataTypeStr=fixdt(0, 8, 7)  OutDataTypeStr=fixdt(0, 16, 7)  SampleTime=1
  cfblk16_out1bypassMux : MultiPortSwitch  DataPortOrder=Zero-based contiguous  Inputs=2  zeroidx=on  OutDataTypeStr=fixdt(0, 16, 7)  SampleTime=1  SaturateOnIntegerOverflow=off  InputSameDT=off
  emi_91_bypass : UnitDelay  InitialCondition="fi(0,0,16,7,\"hex\",\"0000\")"  SampleTime=1
  emi_91 : Outport  SampleTime=1  InitialOutput=0
  wires:
  Action Port/1 -> cfblk16_out1bypassMux/1
  emi_90/1 -> cfblk16/1
  cfblk16/1 -> cfblk16_out1bypassMux/3
  cfblk16_out1bypassMux/1 -> emi_91_bypass/1, emi_91/1
  emi_91_bypass/1 -> cfblk16_out1bypassMux/2

== system gm_sampleModel61706_pp_36_1_sub/Subsystem/cfblk161 ==
  emi_98 : Inport  OutDataTypeStr=uint8  PortDimensions=1  SampleTime=1
  Action Port : Inport  Port=2  OutDataTypeStr=boolean  SampleTime=1
  Reshape : Reshape
  cfblk161_out1bypassMux : MultiPortSwitch  DataPortOrder=Zero-based contiguous  Inputs=2  zeroidx=on  OutDataTypeStr=uint8  SampleTime=1  SaturateOnIntegerOverflow=off  InputSameDT=off
  emi_99_bypass : UnitDelay  InitialCondition="fi(0,0,8,0,\"hex\",\"00\")"  SampleTime=1
  emi_99 : Outport  SampleTime=1  InitialOutput=0
  wires:
  Action Port/1 -> cfblk161_out1bypassMux/1
  emi_98/1 -> Reshape/1
  Reshape/1 -> cfblk161_out1bypassMux/3
  cfblk161_out1bypassMux/1 -> emi_99_bypass/1, emi_99/1
  emi_99_bypass/1 -> cfblk161_out1bypassMux/2

== system gm_sampleModel61706_pp_36_1_sub/Subsystem/cfblk162_inst ==
  in1 : Inport  OutDataTypeStr=uint8  SampleTime=1
  in2 : Inport  Port=2  OutDataTypeStr=uint8  SampleTime=1
  mul_cfblk162_dotp_mulcomp : Product  Inputs=**  OutDataTypeStr=uint8  SampleTime=1
  out1 : Outport  OutDataTypeStr=uint8  SampleTime=1
  wires:
  in1/1 -> mul_cfblk162_dotp_mulcomp/1
  in2/1 -> mul_cfblk162_dotp_mulcomp/2
  mul_cfblk162_dotp_mulcomp/1 -> out1/1

== system gm_sampleModel61706_pp_36_1_sub/Subsystem/cfblk164 ==
  emi_106 : Inport  OutDataTypeStr=uint8  PortDimensions=1  SampleTime=1
  Action Port : Inport  Port=2  OutDataTypeStr=boolean  SampleTime=1
  cfblk164 : Sum  Inputs=+
  cfblk164_out1bypassMux : MultiPortSwitch  DataPortOrder=Zero-based contiguous  Inputs=2  zeroidx=on  OutDataTypeStr=uint8  SampleTime=1  SaturateOnIntegerOverflow=off  InputSameDT=off
  emi_107_bypass : UnitDelay  InitialCondition="fi(0,0,8,0,\"hex\",\"00\")"  SampleTime=1
  emi_107 : Outport  SampleTime=1  InitialOutput=0
  wires:
  Action Port/1 -> cfblk164_out1bypassMux/1
  emi_106/1 -> cfblk164/1
  cfblk164/1 -> cfblk164_out1bypassMux/3
  cfblk164_out1bypassMux/1 -> emi_107_bypass/1, emi_107/1
  emi_107_bypass/1 -> cfblk164_out1bypassMux/2

== system gm_sampleModel61706_pp_36_1_sub/Subsystem/cfblk172_inst ==
  in1 : Inport  OutDataTypeStr=uint8  SampleTime=1
  in2 : Inport  Port=2  OutDataTypeStr=uint8  SampleTime=1
  mul_cfblk172_dotp_mulcomp : Product  Inputs=**  OutDataTypeStr=uint8  SampleTime=1
  out1 : Outport  OutDataTypeStr=uint8  SampleTime=1
  wires:
  in1/1 -> mul_cfblk172_dotp_mulcomp/1
  in2/1 -> mul_cfblk172_dotp_mulcomp/2
  mul_cfblk172_dotp_mulcomp/1 -> out1/1

== system gm_sampleModel61706_pp_36_1_sub/Subsystem/cfblk174 ==
  emi_122 : Inport  OutDataTypeStr=uint8  PortDimensions=1  SampleTime=1
  Action Port : Inport  Port=2  OutDataTypeStr=boolean  SampleTime=1
  cfblk174 : Sum  Inputs=+
  cfblk174_out1bypassMux : MultiPortSwitch  DataPortOrder=Zero-based contiguous  Inputs=2  zeroidx=on  OutDataTypeStr=uint8  SampleTime=1  SaturateOnIntegerOverflow=off  InputSameDT=off
  emi_123_bypass : UnitDelay  InitialCondition="fi(0,0,8,0,\"hex\",\"00\")"  SampleTime=1
  emi_123 : Outport  SampleTime=1  InitialOutput=0
  wires:
  Action Port/1 -> cfblk174_out1bypassMux/1
  emi_122/1 -> cfblk174/1
  cfblk174/1 -> cfblk174_out1bypassMux/3
  cfblk174_out1bypassMux/1 -> emi_123_bypass/1, emi_123/1
  emi_123_bypass/1 -> cfblk174_out1bypassMux/2

== system gm_sampleModel61706_pp_36_1_sub/Subsystem/cfblk176 ==
  emi_187 : Inport  OutDataTypeStr=uint8  PortDimensions=1  SampleTime=1
  Action Port : Inport  Port=2  OutDataTypeStr=boolean  SampleTime=1
  cfblk176 : Abs  SampleTime=1  OutDataTypeStr=uint8  SaturateOnIntegerOverflow=off
  cfblk176_out1bypassMux : MultiPortSwitch  DataPortOrder=Zero-based contiguous  Inputs=2  zeroidx=on  OutDataTypeStr=uint8  SampleTime=1  SaturateOnIntegerOverflow=off  InputSameDT=off
  emi_188_bypass : UnitDelay  InitialCondition="fi(0,0,8,0,\"hex\",\"00\")"  SampleTime=1
  emi_188 : Outport  SampleTime=1  InitialOutput=0
  wires:
  Action Port/1 -> cfblk176_out1bypassMux/1
  emi_187/1 -> cfblk176/1
  cfblk176/1 -> cfblk176_out1bypassMux/3
  cfblk176_out1bypassMux/1 -> emi_188_bypass/1, emi_188/1
  emi_188_bypass/1 -> cfblk176_out1bypassMux/2

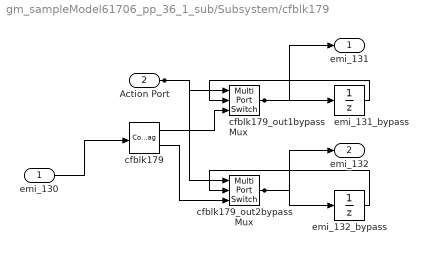
== system gm_sampleModel61706_pp_36_1_sub/Subsystem/cfblk179 ==
  emi_130 : Inport  OutDataTypeStr=uint8  PortDimensions=1  SampleTime=1
  Action Port : Inport  Port=2  OutDataTypeStr=boolean  SampleTime=1
  cfblk179 : ComplexToRealImag  SampleTime=1
  cfblk179_out1bypassMux : MultiPortSwitch  DataPortOrder=Zero-based contiguous  Inputs=2  zeroidx=on  OutDataTypeStr=uint8  SampleTime=1  SaturateOnIntegerOverflow=off  InputSameDT=off
  cfblk179_out2bypassMux : MultiPortSwitch  DataPortOrder=Zero-based contiguous  Inputs=2  zeroidx=on  OutDataTypeStr=uint8  SampleTime=1  SaturateOnIntegerOverflow=off  InputSameDT=off
  emi_131_bypass : UnitDelay  InitialCondition="fi(0,0,8,0,\"hex\",\"00\")"  SampleTime=1
  emi_132_bypass : UnitDelay  InitialCondition="fi(0,0,8,0,\"hex\",\"00\")"  SampleTime=1
  emi_131 : Outport  SampleTime=1  InitialOutput=0
  emi_132 : Outport  Port=2  SampleTime=1  InitialOutput=0
  wires:
  Action Port/1 -> cfblk179_out2bypassMux/1, cfblk179_out1bypassMux/1
  emi_130/1 -> cfblk179/1
  cfblk179/1 -> cfblk179_out1bypassMux/3
  cfblk179/2 -> cfblk179_out2bypassMux/3
  cfblk179_out1bypassMux/1 -> emi_131_bypass/1, emi_131/1
  emi_131_bypass/1 -> cfblk179_out1bypassMux/2
  cfblk179_out2bypassMux/1 -> emi_132_bypass/1, emi_132/1
  emi_132_bypass/1 -> cfblk179_out2bypassMux/2

== system gm_sampleModel61706_pp_36_1_sub/Subsystem/cfblk182 ==
  u : Inport  OutDataTypeStr=uint8  SampleTime=1
  FixPt Constant : Constant  DisableCoverage=on  OutDataTypeStr=Inherit: Inherit via back propagation  SampleTime=-1
  FixPt Data Type Duplicate : DataTypeDuplicate  DisableCoverage=on  NumInputPorts=3
  FixPt Sum1 : Sum  OutDataTypeStr=Inherit: Inherit via back propagation  InputSameDT=on  LockScale=on
  y : Outport  SampleTime=1
  wires:
  u/1 -> FixPt Sum1/1, FixPt Data Type Duplicate/2
  FixPt Constant/1 -> FixPt Sum1/2, FixPt Data Type Duplicate/3
  FixPt Sum1/1 -> FixPt Data Type Duplicate/1, y/1

== system gm_sampleModel61706_pp_36_1_sub/Subsystem/cfblk188 ==
  In1 : Inport  OutDataTypeStr=uint8  PortDimensions=1  SampleTime=1
  Out1 : Outport  SampleTime=1  InitialOutput=[0]
  wires:
  In1/1 -> Out1/1

== system gm_sampleModel61706_pp_36_1_sub/Subsystem/cfblk189 ==
  In1 : Inport  OutDataTypeStr=uint8  PortDimensions=1  SampleTime=1
  Out1 : Outport  SampleTime=1  InitialOutput=[0]
  wires:
  In1/1 -> Out1/1

== system gm_sampleModel61706_pp_36_1_sub/Subsystem/cfblk197 ==
  emi_267 : Inport  OutDataTypeStr=uint8  PortDimensions=1  SampleTime=1
  Action Port : Inport  Port=2  OutDataTypeStr=boolean  SampleTime=1
  cfblk197 : Subsystem
      settings: MinAlgLoopOccurrences=on
  emi_268 : Outport  SampleTime=1  InitialOutput=0
  wires:
  Action Port/1 -> cfblk197/Enable
  emi_267/1 -> cfblk197/1(in0)
  cfblk197/1(out0) -> emi_268/1

== system gm_sampleModel61706_pp_36_1_sub/Subsystem/cfblk2 ==
  u : Inport  OutDataTypeStr=uint8  SampleTime=1
  Compare : RelationalOperator  Operator=<=  OutDataTypeStr=fixdt(0, 8)
  Constant : Constant  DisableCoverage=on  Value=const  OutDataTypeStr=Inherit: Inherit via back propagation  SampleTime=-1
  y : Outport  SampleTime=1
  wires:
  u/1 -> Compare/1
  Compare/1 -> y/1
  Constant/1 -> Compare/2

== system gm_sampleModel61706_pp_36_1_sub/Subsystem/cfblk200 ==
  emi_219 : Inport  OutDataTypeStr=uint8  PortDimensions=1  SampleTime=1
  Action Port : Inport  Port=2  OutDataTypeStr=boolean  SampleTime=1
  cfblk200 : Subsystem
      settings: MinAlgLoopOccurrences=on
  emi_220 : Outport  SampleTime=1  InitialOutput=0
  wires:
  Action Port/1 -> cfblk200/Enable
  emi_219/1 -> cfblk200/1(in0)
  cfblk200/1(out0) -> emi_220/1

== system gm_sampleModel61706_pp_36_1_sub/Subsystem/cfblk218 ==
  emi_139 : Inport  OutDataTypeStr=uint8  PortDimensions=1  SampleTime=1
  Action Port : Inport  Port=2  OutDataTypeStr=boolean  SampleTime=1
  cfblk218 : DataTypeConversion  OutDataTypeStr=fixdt(0,8,0)
  cfblk218_out1bypassMux : MultiPortSwitch  DataPortOrder=Zero-based contiguous  Inputs=2  zeroidx=on  OutDataTypeStr=uint8  SampleTime=1  SaturateOnIntegerOverflow=off  InputSameDT=off
  emi_140_bypass : UnitDelay  InitialCondition="fi(0,0,8,0,\"hex\",\"00\")"  SampleTime=1
  emi_140 : Outport  SampleTime=1  InitialOutput=0
  wires:
  Action Port/1 -> cfblk218_out1bypassMux/1
  emi_139/1 -> cfblk218/1
  cfblk218/1 -> cfblk218_out1bypassMux/3
  cfblk218_out1bypassMux/1 -> emi_140_bypass/1, emi_140/1
  emi_140_bypass/1 -> cfblk218_out1bypassMux/2

== system gm_sampleModel61706_pp_36_1_sub/Subsystem/cfblk28 ==
  emi_66 : Inport  OutDataTypeStr=uint8  PortDimensions=1  SampleTime=1
  Action Port : Inport  Port=2  OutDataTypeStr=boolean  SampleTime=1
  cfblk28 : Subsystem  mask(Real World Value Increment){}
      mask help: Simulink:masks:RealWorldValueIncrement_MD
      mask Display: disp('V++')
  cfblk28_out1bypassMux : MultiPortSwitch  DataPortOrder=Zero-based contiguous  Inputs=2  zeroidx=on  OutDataTypeStr=uint8  SampleTime=1  SaturateOnIntegerOverflow=off  InputSameDT=off
  emi_67_bypass : UnitDelay  InitialCondition="fi(0,0,8,0,\"hex\",\"00\")"  SampleTime=1
  emi_67 : Outport  SampleTime=1  InitialOutput=0
  wires:
  Action Port/1 -> cfblk28_out1bypassMux/1
  emi_66/1 -> cfblk28/1(u)
  cfblk28/1(y) -> cfblk28_out1bypassMux/3
  cfblk28_out1bypassMux/1 -> emi_67_bypass/1, emi_67/1
  emi_67_bypass/1 -> cfblk28_out1bypassMux/2

== system gm_sampleModel61706_pp_36_1_sub/Subsystem/cfblk3 ==
  emi_155 : Inport  OutDataTypeStr=uint8  PortDimensions=1  SampleTime=1
  Action Port : Inport  Port=2  OutDataTypeStr=boolean  SampleTime=1
  cfblk3 : hdlsllib/Logic and Bit Operations/Interval Test  IntervalClosedRight=on  uplimit=0.5  IntervalClosedLeft=on  lowlimit=-0.5  OutDataTypeStr=uint8
  cfblk3_out1bypassMux : MultiPortSwitch  DataPortOrder=Zero-based contiguous  Inputs=2  zeroidx=on  OutDataTypeStr=uint8  SampleTime=1  SaturateOnIntegerOverflow=off  InputSameDT=off
  emi_156_bypass : UnitDelay  InitialCondition="fi(0,0,8,0,\"hex\",\"00\")"  SampleTime=1
  emi_156 : Outport  SampleTime=1  InitialOutput=0
  wires:
  Action Port/1 -> cfblk3_out1bypassMux/1
  emi_155/1 -> cfblk3/1
  cfblk3/1 -> cfblk3_out1bypassMux/3
  cfblk3_out1bypassMux/1 -> emi_156_bypass/1, emi_156/1
  emi_156_bypass/1 -> cfblk3_out1bypassMux/2

== system gm_sampleModel61706_pp_36_1_sub/Subsystem/cfblk32 ==
  emi_163 : Inport  OutDataTypeStr=fixdt(0, 16, 7)  PortDimensions=1  SampleTime=1
  Action Port : Inport  Port=2  OutDataTypeStr=boolean  SampleTime=1
  cfblk32 : MinMax
  cfblk32_out1bypassMux : MultiPortSwitch  DataPortOrder=Zero-based contiguous  Inputs=2  zeroidx=on  OutDataTypeStr=fixdt(0, 16, 7)  SampleTime=1  SaturateOnIntegerOverflow=off  InputSameDT=off
  emi_164_bypass : UnitDelay  InitialCondition="fi(0,0,16,7,\"hex\",\"0000\")"  SampleTime=1
  emi_164 : Outport  SampleTime=1  InitialOutput=0
  wires:
  Action Port/1 -> cfblk32_out1bypassMux/1
  emi_163/1 -> cfblk32/1
  cfblk32/1 -> cfblk32_out1bypassMux/3
  cfblk32_out1bypassMux/1 -> emi_164_bypass/1, emi_164/1
  emi_164_bypass/1 -> cfblk32_out1bypassMux/2

== system gm_sampleModel61706_pp_36_1_sub/Subsystem/cfblk37 ==
  emi_171 : Inport  OutDataTypeStr=uint8  PortDimensions=1  SampleTime=1
  Action Port : Inport  Port=2  OutDataTypeStr=boolean  SampleTime=1
  cfblk37 : Subsystem  mask(Real World Value Increment){}
      mask help: Simulink:masks:RealWorldValueIncrement_MD
      mask Display: disp('V++')
  cfblk37_out1bypassMux : MultiPortSwitch  DataPortOrder=Zero-based contiguous  Inputs=2  zeroidx=on  OutDataTypeStr=uint8  SampleTime=1  SaturateOnIntegerOverflow=off  InputSameDT=off
  emi_172_bypass : UnitDelay  InitialCondition="fi(0,0,8,0,\"hex\",\"00\")"  SampleTime=1
  emi_172 : Outport  SampleTime=1  InitialOutput=0
  wires:
  Action Port/1 -> cfblk37_out1bypassMux/1
  emi_171/1 -> cfblk37/1(u)
  cfblk37/1(y) -> cfblk37_out1bypassMux/3
  cfblk37_out1bypassMux/1 -> emi_172_bypass/1, emi_172/1
  emi_172_bypass/1 -> cfblk37_out1bypassMux/2
